simulink model "point_2"  (R2022a)
settings: Solver=VariableStepAuto  StartTime=0.0  StopTime=T_sim  RelTol=1e-3
values from neighbouring files (symbols this model uses):
  A = [-1.2822  0      0.98     0 ... (first row only)    [main.m]    (also in main_cessna.m = [-1.2822 0 0.98 0)
  B = [-0.3 ... (first row only)    [main.m]    (also in main_cessna.m)
  C = [0       1      0  0 ... (first row only)    [main.m]    (also in main_cessna.m = [0 1 0 0)
  C_states = eye(length(A))    [main.m]    (also in main_cessna.m = eye(4))
  D_states = zeros(length(B), 1)    [main.m]
  sysd = c2d(sys,T_sampling)    [main.m]
  T_sampling = 2*pi/omega_sampling    [main.m]
  u_max = deg2rad(15)    [main.m]
  u_min = deg2rad(-15)    [main.m]
  x0 = [deg2rad(0) deg2rad(15) 0 -300]    [main.m]    (also in main_cessna.m = [0 0 0 5000])
  x_ref = [0 0 0 0]    [main.m]
undefined symbols (not defined in the file or in its folder): k_LQ4, Klqr_d
settings Model: Creator=PaoloA  LastModifiedBy=g_mor
settings DebuggingCC: UnconnectedInputMsg=warning  UnconnectedOutputMsg=warning  UnconnectedLineMsg=warning
settings RTWCC: DLArmComputeVersion=19.05

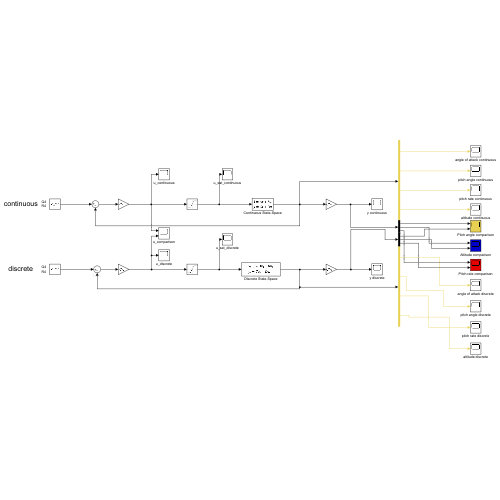
[thumbnail: Simulink's stored preview of the top-level diagram]
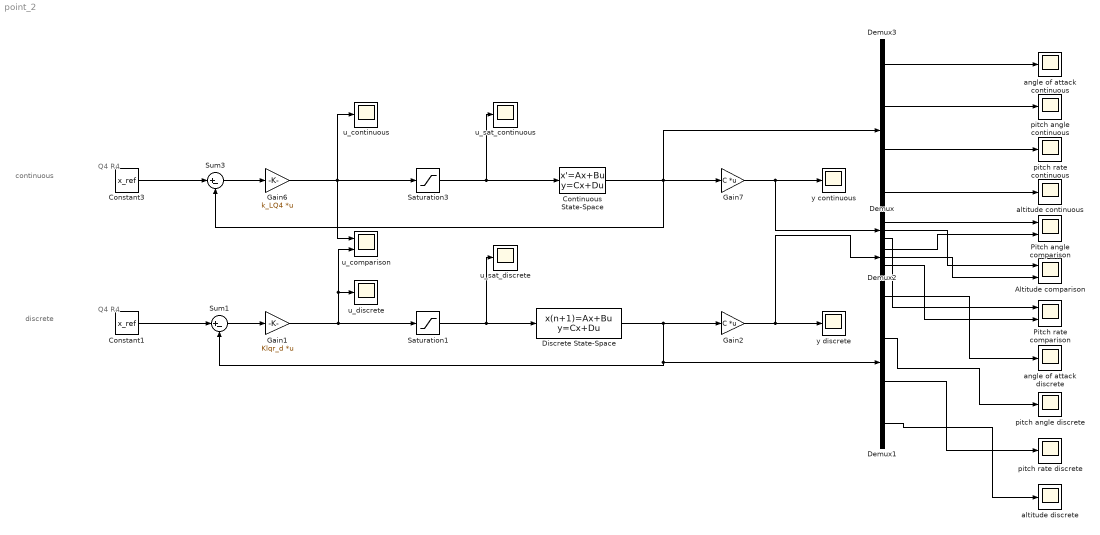
== system point_2 ==
  note: Q4
      | R4
  note: Q4
      | R4
  note: continuous
  note: discrete
  Altitude comparison : Scope  NumInputPorts=2
  Constant1 : Constant  Value=x_ref
  Constant3 : Constant  Value=x_ref
  Continuous State-Space : StateSpace  A=A  B=B  C=C_states  D=D_states  InitialCondition=x0
  Demux : Demux  Outputs=3
  Demux1 : Demux
  Demux2 : Demux  Outputs=3
  Demux3 : Demux
  Discrete State-Space : DiscreteStateSpace  A=sysd.A  B=sysd.B  C=C_states  D=D_states  InitialCondition=x0  SampleTime=T_sampling
  Gain1 : Gain  Gain=Klqr_d  Multiplication=Matrix(K*u)
  Gain2 : Gain  Gain=C  Multiplication=Matrix(K*u)
  Gain6 : Gain  Gain=k_LQ4  Multiplication=Matrix(K*u)
  Gain7 : Gain  Gain=C  Multiplication=Matrix(K*u)
  Pitch angle comparison : Scope  NumInputPorts=2
  Pitch rate comparison : Scope  NumInputPorts=2
  Saturation1 : Saturate  UpperLimit=u_max  LowerLimit=u_min
  Saturation3 : Saturate  UpperLimit=u_max  LowerLimit=u_min
  Sum1 : Sum  Inputs=|+-
  Sum3 : Sum  Inputs=|+-
  altitude continuous : Scope
  altitude discrete : Scope
  angle of attack continuous : Scope
  angle of attack discrete : Scope
  pitch angle continuous : Scope
  pitch angle discrete : Scope
  pitch rate continuous : Scope
  pitch rate discrete : Scope
  u_comparison : Scope  NumInputPorts=2
  u_continuous : Scope
  u_discrete : Scope
  u_sat_continuous : Scope
  u_sat_discrete : Scope
  y continuous : Scope
  y discrete : Scope
  wires:
  Gain6/1 -> u_comparison/1, u_continuous/1, Saturation3/1
  Constant3/1 -> Sum3/1
  Sum3/1 -> Gain6/1
  Saturation3/1 -> u_sat_continuous/1, Continuous State-Space/1
  Continuous State-Space/1 -> Sum3/2, Demux3/1, Gain7/1
  Demux3/2 -> pitch angle continuous/1
  Demux3/1 -> angle of attack continuous/1
  Demux3/3 -> pitch rate continuous/1
  Demux3/4 -> altitude continuous/1
  Gain7/1 -> Demux/1, y continuous/1
  Gain2/1 -> Demux2/1, y discrete/1
  Demux1/2 -> pitch angle discrete/1
  Demux1/4 -> altitude discrete/1
  Gain1/1 -> u_comparison/2, u_discrete/1, Saturation1/1
  Demux1/1 -> angle of attack discrete/1
  Discrete State-Space/1 -> Sum1/2, Demux1/1, Gain2/1
  Saturation1/1 -> Discrete State-Space/1, u_sat_discrete/1
  Constant1/1 -> Sum1/1
  Demux1/3 -> pitch rate discrete/1
  Sum1/1 -> Gain1/1
  Demux/1 -> Pitch angle comparison/1
  Demux/2 -> Altitude comparison/1
  Demux/3 -> Pitch rate comparison/1
  Demux2/1 -> Pitch angle comparison/2
  Demux2/2 -> Altitude comparison/2
  Demux2/3 -> Pitch rate comparison/2
